simulink model "magField_test"  (R2018b)
settings: Solver=VariableStepAuto  StartTime=0.0  StopTime=10.0  RelTol=1e-3
values from neighbouring files (symbols this model uses):
  state = [r;v;q;w]    [magField_test_init.m]
  utc_sec = 1557355288    [magField_test_init.m]
libraries: magField_lib x1, time_Lib x1
settings Model: Creator=Kate  LastModifiedBy=Kate

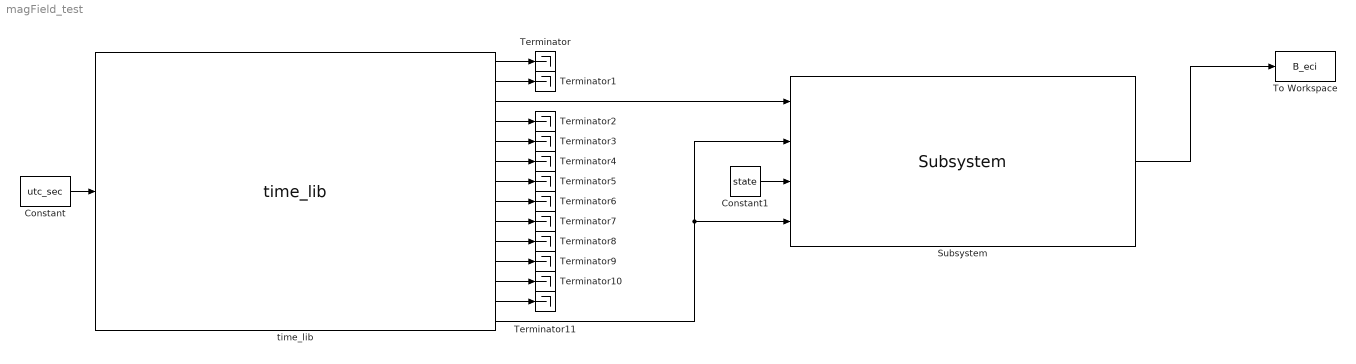
== system magField_test ==
  Constant : Constant  Value=utc_sec
  Constant1 : Constant  Value=state
  Subsystem : magField_lib/Subsystem  SystemSampleTime=-1
  Terminator{,1..11} (12 alike) : Terminator
  To Workspace : ToWorkspace  VariableName=B_eci  SaveFormat=Timeseries  SampleTime=-1
  "time_lib " : time_Lib/time_lib    SystemSampleTime=-1
  wires:
  "time_lib "/1 -> Terminator/1
  "time_lib "/2 -> Terminator1/1
  "time_lib "/4 -> Terminator2/1
  "time_lib "/5 -> Terminator3/1
  "time_lib "/6 -> Terminator4/1
  "time_lib "/7 -> Terminator5/1
  "time_lib "/8 -> Terminator6/1
  "time_lib "/9 -> Terminator7/1
  "time_lib "/10 -> Terminator8/1
  "time_lib "/11 -> Terminator9/1
  "time_lib "/12 -> Terminator10/1
  "time_lib "/13 -> Terminator11/1
  Subsystem/1 -> To Workspace/1
  Constant/1 -> "time_lib "/1
  "time_lib "/3 -> Subsystem/1
  "time_lib "/14 -> Subsystem/2, Subsystem/4
  Constant1/1 -> Subsystem/3
